simulink model "rectgen_mod"  (R2020b)
settings: Solver=VariableStepAuto  StartTime=0.0  StopTime=10.0  RelTol=1e-3
values from neighbouring files (symbols this model uses):
  a1 = R*C1    (= 0.05185)    [PT3_dat.m]    (also in Regler_dat.m = 0.08; UE7_1.m = 0.08; fun_RLC_Euler.m = 2*D/w0)
  a2 = L*(C1+C2)    (= 0.000408)    [PT3_dat.m]    (also in Regler_dat.m = 0.04; UE7_1.m = 0.04; fun_RLC_Euler.m = 1/w0^2)
  a3 = R*L*C1*C2    (= 1.23403e-05)    [PT3_dat.m]
  s1 = 0.9    [PT3_dat.m]
  s2 = 0.1    [PT3_dat.m]
settings Model: Creator=Sinh  LastModifiedBy=Sinh

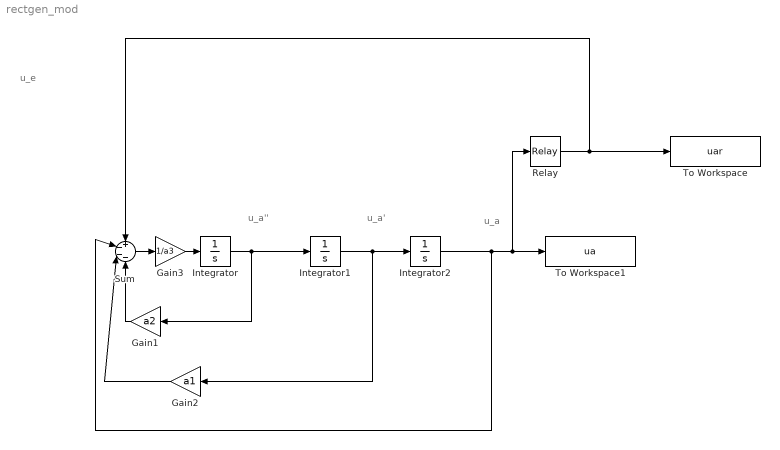
== system rectgen_mod ==
  note: u_a
  note: u_a'
  note: u_a''
  note: u_e
  Gain1 : Gain  Gain=a2
  Gain2 : Gain  Gain=a1
  Gain3 : Gain  Gain=1/a3
  Integrator : Integrator
  Integrator1 : Integrator
  Integrator2 : Integrator
  Relay : Relay  OnSwitchValue=s1  OffSwitchValue=s2  OnOutputValue=ylow  OffOutputValue=yhigh
  Sum : Sum  Inputs=+---
  To Workspace : ToWorkspace  VariableName=uar  SampleTime=-1
  To Workspace1 : ToWorkspace  VariableName=ua  SampleTime=-1
  wires:
  Integrator1/1 -> Gain2/1, Integrator2/1
  Gain1/1 -> Sum/4
  Integrator/1 -> Gain1/1, Integrator1/1
  Gain2/1 -> Sum/3
  Integrator2/1 -> Sum/2, Relay/1, To Workspace1/1
  Sum/1 -> Gain3/1
  Gain3/1 -> Integrator/1
  Relay/1 -> To Workspace/1, Sum/1
